simulink subsystem "Final_Project_DistHold_attempt_20260602_205044"  (R2024a)
settings: Solver=VariableStepAuto  StartTime=0.0  StopTime=10.0  RelTol=1e-3
values from neighbouring files (symbols this model uses):
  D = hypot(Ep(:,1)-Tp(:,1)',Ep(:,2)-Tp(:,2)')    [pp_compare_stage.m]    (also in pp_diag_path.m; pp_t09_clear.m = hypot(Ep(:,1)-Tperim(:,1)', Ep(:,2)-Tperim(:,2)'); pp_tune2.m)
undefined symbols (not defined in the file or in its folder): DiscIntNeverNeededParam, waypoint_const
libraries: CarMaker4SL x83, simulink x2
(part 5 of 5)

== matlab function Final_Project_DistHold_attempt_20260602_205044/Parking_system/MATLAB Function6 ==
  data: ego_x input; desired_ax output; ego_y input; ego_yaw input; ego_v input; start_point input; finish_point input; goal_yaw input; occ_map input; steer_fl output; steer_fr output; selector_ctrl output
function [desired_ax, steer_fl, steer_fr, selector_ctrl] = Parking(ego_x, ego_y, ego_yaw, ego_v, start_point, finish_point, goal_yaw, occ_map)
%PARKING  Self-contained version of the "MATLAB Function" block.
%   Source model : Models/Day4_5/Day4_5_Scenario_1.slx
%   Block path   : CarMaker/Subsystem/Day4 & 5/Scenario 1/MATLAB Function
%
%   The block body only calls the pp_* helper; this file additionally
%   bundles every pp_*.m it transitively depends on as local functions,
%   so it runs standalone without dev/day4_5/pp_*.m on the MATLAB path.
%
%   Bundled depQendencies (15): pp_parking, pp_ackermann, pp_angdiff, pp_axle_from_fr1, pp_cfg, pp_collision, pp_grid2world, pp_hybrid_astar, pp_pt_in_quad, pp_rect_corners, pp_reedsshepp, pp_rs_paths, pp_rs_sample, pp_track, pp_world2grid
[desired_ax, steer_fl, steer_fr, selector_ctrl] = pp_parking(ego_x, ego_y, ego_yaw, ego_v, start_point, finish_point, goal_yaw, occ_map);
end

% ========================================================================
%  Local dependency functions (bundled verbatim from dev/day4_5/pp_*.m).
%  Do not edit here; edit the pp_*.m sources and re-bundle.
% ========================================================================

function [desired_ax, steer_fl, steer_fr, selector_ctrl] = pp_parking(ego_x, ego_y, ego_yaw, ego_v, start_point, finish_point, goal_yaw, occ_map) %#ok<INUSD>
%#codegen
% PP_PARKING  Full precise-parking controller (M10 integration).
%   Supervisor: INIT -> PLAN (Hybrid A*+RS, once) -> TRACK (pure pursuit) ->
%   CORRECT (a few committed Reeds-Shepp corrective rounds, each tracked by
%   pp_track) -> PARKED. Using committed RS paths (fixed cusps) instead of
%   per-step RS feedback avoids gear-shift chatter on the real plant.
%   Gear FSM shifts only when (nearly) stopped. Longitudinal command is in the
%   DRIVING (gear) direction (CarMaker AccelCtrl convention) with an over-speed
%   guard. Ackermann splits the steer into L/R wheels.
%
%   Inputs (Car.Fr1 = rear-bumper center): ego_x,ego_y[m], ego_yaw, ego_v[m/s],
%   finish_point=[x y] (rear bumper), goal_yaw[rad], occ_map. start_point unused.
cfg = pp_cfg(); d_r = cfg.d_r; L = cfg.wheelbase; tw = cfg.track_f; MAXP = cfg.max_path;

persistent state PX PY PDIR NP seg gear replan nround
if isempty(state)
    state = uint8(0);
    PX = zeros(MAXP,1); PY = zeros(MAXP,1); PDIR = zeros(MAXP,1);
    NP = 0; seg = 1; gear = cfg.GEAR_P; replan = false; nround = 0;
end

[ex, ey] = pp_axle_from_fr1(ego_x, ego_y, ego_yaw, d_r); eth = ego_yaw;
gth = goal_yaw;
[gx, gy] = pp_axle_from_fr1(finish_point(1), finish_point(2), gth, d_r);

delta = 0.0; v_des = 0.0; hold = false;

switch state
    case uint8(0)                                       % INIT
        state = uint8(1); hold = true;

    case uint8(1)                                       % PLAN (one heavy step)
        [px, py, ~, pdir, np, ok] = pp_hybrid_astar(ex, ey, eth, gx, gy, gth, occ_map);
        if ok
            PX = px; PY = py; PDIR = pdir; NP = np; seg = 1; state = uint8(2);
        else
            state = uint8(4);
        end
        hold = true;

    case uint8(2)                                       % TRACK main path
        [delta, v_des, seg, done] = pp_track(ex, ey, eth, ego_v, PX, PY, PDIR, NP, seg, cfg);
        if done, state = uint8(3); replan = true; nround = 0; end

    case uint8(3)                                       % CORRECT (committed RS rounds)
        if replan
            [Tr, sLr, ~, okr] = pp_reedsshepp(ex, ey, eth, gx, gy, gth, cfg.Rmin);
            if okr
                [rx, ry, ~, rdir, rns] = pp_rs_sample(ex, ey, eth, Tr, sLr, cfg.Rmin, cfg.ds, MAXP);
                if rns >= 2
                    PX = rx; PY = ry; PDIR = rdir; NP = rns; seg = 1;
                    replan = false; nround = nround + 1;
                else
                    state = uint8(4);
                end
            else
                state = uint8(4);
            end
        end
        if state == uint8(3)
            [delta, v_des, seg, done] = pp_track(ex, ey, eth, ego_v, PX, PY, PDIR, NP, seg, cfg);
            if done
                if (hypot(gx-ex, gy-ey) < cfg.align_pos && abs(pp_angdiff(eth,gth)) < cfg.align_yaw) ...
                        || nround >= cfg.max_rounds
                    state = uint8(4);
                else
                    replan = true;                      % next committed round
                end
            end
        end

    otherwise                                           % PARKED
        hold = true;
end
if state == uint8(4), hold = true; end

% --- outputs: gear FSM + longitudinal (driving-dir) + Ackermann ---
if hold
    selector_ctrl = cfg.GEAR_P;
    desired_ax    = -1.0;
    steer_fl      = 0.0; steer_fr = 0.0;
else
    if abs(ego_v) < cfg.v_stop                          % shift only when ~stopped
        if v_des > 0.02
            gear = cfg.GEAR_D;
        elseif v_des < -0.02
            gear = cfg.GEAR_R;
        end
    end
    selector_ctrl = gear;
    % CarMaker AccelCtrl.DesiredAx = GEAR-DIRECTION acceleration demand (CONFIRMED by
    % per-gear regression of the logs: in D +DesiredAx -> +x accel (slope +0.84); in R
    % +DesiredAx -> -x accel (slope -0.90)). So +DesiredAx = gas in the CURRENT GEAR
    % direction (forward in D, BACKWARD in R); -DesiredAx = brake. PRIMARY control is this
    % gear-direction speed regulation toward |v_des|, tracked by the vehicle's AccelCtrl PI
    % (tuned in the .car: higher i compensates the reverse idle-creep). Reverse uses a LOW
    % target speed (cfg.v_rev). The over-target branch is only a SAFETY NET (large margin)
    % in case the PI lags -- it should rarely fire once the PI holds the low reverse speed.
    if gear == cfg.GEAR_R, gdir = -1.0; else, gdir = 1.0; end
    v_drive = gdir*ego_v;                                  % speed in the gear (driving) direction
    desired_ax = cfg.kp_v*(abs(v_des) - v_drive);         % + = gas (gear dir), - = brake
    desired_ax = max(min(desired_ax, cfg.ax_max), -cfg.ax_max);
    if v_drive > cfg.v_emax                                % SAFETY NET: genuine runaway only (PI now
        desired_ax = -cfg.ax_brake;                       % regulates normal speed; no mid-maneuver stops)
    end
    [steer_fl, steer_fr] = pp_ackermann(delta, L, tw);
end
end

function [dL, dR] = pp_ackermann(delta, L, tw)
%#codegen
% PP_ACKERMANN  Left/right front road-wheel angles from a single bicycle steer.
%   delta : bicycle (center) steer angle [rad]; L : wheelbase; tw : front track.
%   Inner wheel steers more than the outer (true Ackermann geometry).
if abs(delta) < 1e-4
    dL = 0.0; dR = 0.0;
    return;
end
R  = L / tan(delta);            % signed turn radius at rear-axle center (+ = left)
dL = atan(L / (R - tw/2));      % left  front wheel
dR = atan(L / (R + tw/2));      % right front wheel
end

function d = pp_angdiff(a, b)
%#codegen
% PP_ANGDIFF  Smallest signed angle a-b wrapped to [-pi, pi].
d = mod(a - b + pi, 2*pi) - pi;
end

function [xa, ya] = pp_axle_from_fr1(x, y, yaw, d_r)
%#codegen
% PP_AXLE_FROM_FR1  Rear-axle position from Fr1 (rear-bumper) pose.
%   Rear axle sits d_r ahead of Fr1 along the heading.
xa = x + d_r*cos(yaw);
ya = y + d_r*sin(yaw);
end

function cfg = pp_cfg()
%#codegen
% PP_CFG  Configuration for the Day4/5 precise-parking controller (Kia_EV6).
%   Geometry from Data/Vehicle/Kia_EV6 (Vehicle.OuterSkin & wheel positions).
%
%   Pose convention (CarMaker): Car.Fr1 origin = REAR-BUMPER center on the road,
%   X forward, Y left, yaw = Car.Fr1.rz [rad]. Same convention for the mission
%   goal pose and every obstacle coordinate. Internal planning/tracking uses the
%   REAR AXLE, d_r ahead of Fr1:  rear_axle = Fr1 + d_r*[cos(yaw) sin(yaw)].
%
%   CODEGEN NOTE: build every struct field from LOCAL variables / literals only.
%   Never read a cfg field while still constructing cfg.

% --- local geometry constants (Kia_EV6) -----------------------------------
veh_L     = 4.68;
veh_W     = 1.88;
wheelbase = 2.90;
d_r       = 0.95;
delta_max = 30*pi/180;

% --- vehicle ---------------------------------------------------------------
cfg.veh_L       = veh_L;
cfg.veh_W       = veh_W;
cfg.veh_halfW   = veh_W/2;
cfg.wheelbase   = wheelbase;
cfg.track_f     = 1.624;                  % front track width [m] (wheels at y=+-0.812)
cfg.d_r         = d_r;
cfg.foot_ahead  = veh_L - d_r;            % rear-axle -> front bumper [m] = 3.73
cfg.foot_behind = d_r;                    % rear-axle -> rear bumper  [m] = 0.95
cfg.delta_max   = delta_max;
cfg.Rmin        = wheelbase / tan(delta_max);

% --- obstacle vehicle (IPG_CompanyCar_2018_Blue) ---------------------------
cfg.obs_L       = 4.47;
cfg.obs_W       = 1.97;
cfg.holdout     = 14;                     % pp_obstacles row kept FREE as the parking
                                          %   target (held-out car). 14 = T13. 0 = none.

% --- occupancy grid --------------------------------------------------------
cfg.n           = 200;                    % cells/side (occ_map [200 200]) -- keep 200: EML occ port is fixed
cfg.margin      = 0.30;                   % obstacle footprint safety inflation [m] (buffer for tracking error)
cfg.bounds      = [-5 48 -45.5 6];        % world planning rect [xmin xmax ymin ymax] = lot + NORTH entrance approach
                                          %   (res 53/200=0.265 x 51.5/200=0.258 m)
cfg.lot         = [2 48 -45.5 -3];        % drivable parking-lot rectangle [xmin xmax ymin ymax] (carved FREE by pp_generate_map)
cfg.edge_margin = 0.20;                    % safety margin inset from the drivable-region boundary (lot edges + corridor walls) [m]
cfg.wall_cells  = 1;                      % occupied border-ring thickness [cells]

% --- Hybrid A* planner -----------------------------------------------------
cfg.plan_res    = 0.5;                    % closed-set position resolution [m]
cfg.nxc         = 106;                    % closed-set X bins  ~ (bounds_x)/plan_res = 53/0.5
cfg.nyc         = 103;                    % closed-set Y bins  ~ (bounds_y)/plan_res = 51.5/0.5
cfg.nth         = 72;                     % heading bins (5 deg)
cfg.ds          = 0.6;                    % motion step (arc length) [m]
cfg.n_steer     = 5;                      % steering samples (odd, symmetric)
cfg.max_nodes   = 60000;                  % expansion / node cap
cfg.max_path    = 2000;                   % max stored path points
cfg.pos_tol     = 0.7;                    % planner goal position tol [m] (M9 refines)
cfg.yaw_tol     = 12*pi/180;              % planner goal heading tol [rad]
cfg.w_rev       = 2.0;                    % reverse cost multiplier
cfg.w_switch    = 2.0;                    % direction-change penalty [~m]
cfg.w_steer     = 0.3;                    % steering magnitude penalty
cfg.h_weight    = 1.2;                    % heuristic weight (>=1 speeds search)
cfg.rs_shot_dist = 15.0;                  % try RS one-shot to goal within this dist [m]
cfg.rs_heur_dist = 25.0;                  % use RS (vs Euclidean) heuristic within [m]

% --- M7 path tracking + longitudinal control -------------------------------
cfg.Ld          = 1.5;                    % (legacy) nominal lookahead [m]
cfg.Ld_min      = 0.5;                    % min lookahead (tight low-speed tracking) [m]
cfg.Ld_max      = 1.8;                    % max lookahead [m]
cfg.kld         = 1.2;                    % lookahead gain vs |speed| (Ld = Ld_min + kld*|v|)
cfg.v_fwd       = 1.0;                    % forward cruise speed [m/s] (faster approach)
cfg.v_rev       = 0.2;                    % reverse cruise speed [m/s] (known-good; speed-up revisited separately)
cfg.v_creep     = 0.10;                   % min creep speed while cruising [m/s]
cfg.v_stop      = 0.10;                   % treated as stopped [m/s]
cfg.kp_v        = 0.6;                    % longitudinal P gain (outer speed loop)
cfg.ax_max      = 0.6;                    % accel/brake command limit [m/s^2]
cfg.ax_min      = -1.5;                   % emergency decel/brake limit [m/s^2]
cfg.v_emax      = 1.2;                    % over-speed guard -> emergency brake [m/s]
cfg.v_obrake    = 0.40;                   % SAFETY-NET margin over target -> hard brake [m/s] (PI handles normal regulation)
cfg.ax_brake    = 1.5;                    % safety-net brake demand magnitude [m/s^2] (gear-dir: -ve = brake)
cfg.d_slow      = 5.0;                    % slow-down distance before cusp/goal [m] (weak brake -> decelerate early)
cfg.cusp_reach  = 0.30;                   % distance to register a cusp reached [m]
cfg.goal_reach  = 0.08;                   % path-end position tol [m]
cfg.max_rounds  = 4;                      % max RS corrective rounds in ALIGN (few shifts)

% --- M9 precise pose alignment (Astolfi pose regulation) -------------------
cfg.align_dist  = 3.0;                    % switch to alignment within this dist [m]
cfg.align_pos   = 0.08;                   % alignment done position tol [m]
cfg.align_yaw   = 2*pi/180;               % alignment done heading tol [rad]
cfg.v_align     = 0.3;                    % alignment creep speed [m/s]
cfg.v_align_min = 0.15;                   % min alignment creep speed [m/s]
cfg.kr          = 0.5;                    % Astolfi rho gain (approach)
cfg.ka          = 1.5;                    % Astolfi alpha gain (bearing)
cfg.kb          = -0.5;                   % Astolfi beta gain (final heading, <0)

% --- CarMaker gear selector enum (include/Vehicle.h) -----------------------
cfg.GEAR_P      = -9;
cfg.GEAR_R      = -1;
cfg.GEAR_N      = 0;
cfg.GEAR_D      = 1;
end

function tf = pp_collision(map, x, y, yaw, ahead, behind, halfw, b, n)
%#codegen
% PP_COLLISION  True if the oriented footprint at pose (x,y,yaw) overlaps any
%   occupied cell (map > 0). Pose is the REAR-AXLE reference; the footprint
%   spans [-behind,+ahead] x [-halfw,+halfw]. Scans the footprint bounding box.
c = pp_rect_corners(x, y, yaw, ahead, behind, halfw);
ixv = zeros(1, 4); iyv = zeros(1, 4);
for k = 1:4
    [ixv(k), iyv(k)] = pp_world2grid(c(k,1), c(k,2), b, n);
end
imin = max(min(ixv), 1); imax = min(max(ixv), n);
jmin = max(min(iyv), 1); jmax = min(max(iyv), n);
tf = false;
for ix = imin:imax
    for iy = jmin:jmax
        if map(iy, ix) > 0
            [cx, cy] = pp_grid2world(ix, iy, b, n);
            if pp_pt_in_quad(cx, cy, c)
                tf = true;
                return;
            end
        end
    end
end
end

function [x, y] = pp_grid2world(ix, iy, b, n)
%#codegen
% PP_GRID2WORLD  1-based grid indices -> world coordinates of the CELL CENTER.
%   b = [xmin xmax ymin ymax], n = cells per side.
resx = (b(2) - b(1)) / n;
resy = (b(4) - b(3)) / n;
x = b(1) + (ix - 0.5) * resx;
y = b(3) + (iy - 0.5) * resy;
end

function [px, py, pth, pdir, np, ok] = pp_hybrid_astar(xs, ys, ths, xg, yg, thg, occ_map)
%#codegen
% PP_HYBRID_ASTAR  Hybrid A* parking planner with Reeds-Shepp (REAR-AXLE frame).
%   In : start (xs,ys,ths), goal (xg,yg,thg) [rad], occ_map (n x n, 1=occupied).
%   Out: px,py,pth (max_path x1); pdir (+1 fwd / -1 rev per point); np count; ok.
%   Bicycle fwd/rev primitives + footprint collision; open=min-heap on f=g+h;
%   closed=best-g per (cell,heading). Heuristic = Reeds-Shepp length near goal
%   (Euclidean far). RS one-shot connects to the EXACT goal pose when close.

cfg = pp_cfg();
b = cfg.bounds; n = cfg.n;
plan_res = cfg.plan_res; nxc = cfg.nxc; nyc = cfg.nyc; nth = cfg.nth;
ds = cfg.ds; Lwb = cfg.wheelbase; dmax = cfg.delta_max; Rmin = cfg.Rmin;
ahead = cfg.foot_ahead; behind = cfg.foot_behind; halfw = cfg.veh_halfW;
MAXN = cfg.max_nodes; MAXP = cfg.max_path; ns = cfg.n_steer; hw = cfg.h_weight;
rs_shot = cfg.rs_shot_dist; rs_heur = cfg.rs_heur_dist;
dth_bin = 2*pi/nth;

% steering samples (symmetric about 0)
steer = zeros(1, ns);
for i = 1:ns
    steer(i) = -dmax + (i-1)*(2*dmax/(ns-1));
end

% node + heap + closed storage
NX = zeros(MAXN,1); NY = zeros(MAXN,1); NT = zeros(MAXN,1);
NG = inf(MAXN,1);   NPar = zeros(MAXN,1); NDir = zeros(MAXN,1);
HID = zeros(MAXN,1); HF = inf(MAXN,1); hn = 0;
gbest = inf(nxc, nyc, nth);

% outputs + RS one-shot buffer
px = zeros(MAXP,1); py = zeros(MAXP,1); pth = zeros(MAXP,1); pdir = zeros(MAXP,1);
np = 0; ok = false;
rsx = zeros(MAXP,1); rsy = zeros(MAXP,1); rsth = zeros(MAXP,1); rsdir = zeros(MAXP,1);
rsn = 0; viars = false;

% seed start node
ncount = 1;
NX(1) = xs; NY(1) = ys; NT(1) = ths; NG(1) = 0; NPar(1) = 0; NDir(1) = 0;
six = min(max(floor((xs-b(1))/plan_res)+1,1),nxc);
siy = min(max(floor((ys-b(3))/plan_res)+1,1),nyc);
sit = mod(floor(mod(ths,2*pi)/dth_bin),nth)+1;
gbest(six,siy,sit) = 0;
hn = hn + 1; HID(hn) = 1;
HF(hn) = hw*heur_(xs, ys, ths, xg, yg, thg, Rmin, rs_heur);

goalid = 0; iters = 0;
while hn > 0 && iters < MAXN
    iters = iters + 1;

    % --- heap pop (min f) ---
    cur = HID(1);
    HID(1) = HID(hn); HF(1) = HF(hn); hn = hn - 1;
    hc = 1;
    while true
        hl = 2*hc; hr = 2*hc+1; sm = hc;
        if hl <= hn && HF(hl) < HF(sm), sm = hl; end
        if hr <= hn && HF(hr) < HF(sm), sm = hr; end
        if sm == hc, break; end
        tf = HF(sm); HF(sm) = HF(hc); HF(hc) = tf;
        tk = HID(sm); HID(sm) = HID(hc); HID(hc) = tk;
        hc = sm;
    end

    cx = NX(cur); cy = NY(cur); cth = NT(cur); cg = NG(cur); cdir = NDir(cur);

    % --- tol goal test (fallback) ---
    if abs(cx-xg) < cfg.pos_tol && abs(cy-yg) < cfg.pos_tol && ...
            abs(pp_angdiff(cth,thg)) < cfg.yaw_tol
        goalid = cur; ok = true; break;
    end

    % --- Reeds-Shepp one-shot to exact goal (when close) ---
    if hypot(cx-xg, cy-yg) < rs_shot
        [Tg, segLg, ~, okg] = pp_reedsshepp(cx, cy, cth, xg, yg, thg, Rmin);
        if okg
            [tx, ty, tth, tdir, tn] = pp_rs_sample(cx, cy, cth, Tg, segLg, Rmin, ds, MAXP);
            free = true;
            for sidx = 1:tn
                if pp_collision(occ_map, tx(sidx),ty(sidx),tth(sidx), ahead,behind,halfw, b, n)
                    free = false; break;
                end
            end
            if free
                goalid = cur; ok = true; viars = true; rsn = tn;
                for sidx = 1:tn
                    rsx(sidx)=tx(sidx); rsy(sidx)=ty(sidx); rsth(sidx)=tth(sidx); rsdir(sidx)=tdir(sidx);
                end
                break;
            end
        end
    end

    % --- expand successors (2 directions x ns steers) ---
    for di = 1:2
        if di == 1, dir = 1.0; else, dir = -1.0; end
        sgn = dir*ds;
        for si = 1:ns
            st = steer(si);
            if abs(st) < 1e-6
                nthp = cth;
                nxp = cx + sgn*cos(cth);  nyp = cy + sgn*sin(cth);
                mthp = cth;
                mxp = cx + 0.5*sgn*cos(cth);  myp = cy + 0.5*sgn*sin(cth);
            else
                R = Lwb/tan(st);
                nthp = cth + sgn/R;
                nxp = cx + R*(sin(nthp)-sin(cth));
                nyp = cy - R*(cos(nthp)-cos(cth));
                mthp = cth + 0.5*sgn/R;
                mxp = cx + R*(sin(mthp)-sin(cth));
                myp = cy - R*(cos(mthp)-cos(cth));
            end

            if pp_collision(occ_map, mxp,myp,mthp, ahead,behind,halfw, b, n), continue; end
            if pp_collision(occ_map, nxp,nyp,nthp, ahead,behind,halfw, b, n), continue; end

            stepc = ds;
            if dir < 0, stepc = stepc + ds*(cfg.w_rev-1); end
            if cdir ~= 0 && dir ~= cdir, stepc = stepc + cfg.w_switch; end
            stepc = stepc + cfg.w_steer*abs(st);
            ng = cg + stepc;

            kix = min(max(floor((nxp-b(1))/plan_res)+1,1),nxc);
            kiy = min(max(floor((nyp-b(3))/plan_res)+1,1),nyc);
            kit = mod(floor(mod(nthp,2*pi)/dth_bin),nth)+1;

            if ng < gbest(kix,kiy,kit) && ncount < MAXN
                gbest(kix,kiy,kit) = ng;
                ncount = ncount + 1;
                NX(ncount)=nxp; NY(ncount)=nyp; NT(ncount)=nthp;
                NG(ncount)=ng;  NPar(ncount)=cur; NDir(ncount)=dir;
                fval = ng + hw*heur_(nxp, nyp, nthp, xg, yg, thg, Rmin, rs_heur);
                hn = hn + 1; HID(hn) = ncount; HF(hn) = fval;
                hc = hn;
                while hc > 1
                    hp = floor(hc/2);
                    if HF(hp) <= HF(hc), break; end
                    tf = HF(hp); HF(hp) = HF(hc); HF(hc) = tf;
                    tk = HID(hp); HID(hp) = HID(hc); HID(hc) = tk;
                    hc = hp;
                end
            end
        end
    end
end

% --- reconstruct: Hybrid path (start -> goalid), then append RS one-shot ---
if ok && goalid > 0
    tmpx = zeros(MAXP,1); tmpy = zeros(MAXP,1); tmpt = zeros(MAXP,1); tmpd = zeros(MAXP,1);
    cntr = 0; node = goalid;
    while node ~= 0 && cntr < MAXP
        cntr = cntr + 1;
        tmpx(cntr)=NX(node); tmpy(cntr)=NY(node); tmpt(cntr)=NT(node); tmpd(cntr)=NDir(node);
        node = NPar(node);
    end
    np = cntr;
    for i = 1:cntr
        j = cntr - i + 1;
        px(i)=tmpx(j); py(i)=tmpy(j); pth(i)=tmpt(j); pdir(i)=tmpd(j);
    end
    if cntr >= 2, pdir(1) = pdir(2); end
    if viars
        for sidx = 2:rsn                       % skip RS sample 1 (== node, already added)
            if np >= MAXP, break; end
            np = np + 1;
            px(np)=rsx(sidx); py(np)=rsy(sidx); pth(np)=rsth(sidx); pdir(np)=rsdir(sidx);
        end
    end
end
end

% ===== heuristic: RS length near goal, Euclidean far ======================
function h = heur_(x, y, th, xg, yg, thg, Rmin, rs_heur)
%#codegen
eu = hypot(x-xg, y-yg);
if eu < rs_heur
    [~, ~, Lr, okr] = pp_reedsshepp(x, y, th, xg, yg, thg, Rmin);
    if okr && Lr > eu, h = Lr; else, h = eu; end
else
    h = eu;
end
end

function tf = pp_pt_in_quad(px, py, c)
%#codegen
% PP_PT_IN_QUAD  True if point (px,py) lies inside the convex quad c (4-by-2).
%   Winding-agnostic: inside iff the point is on the same side of all 4 edges.
s = zeros(1, 4);
for k = 1:4
    k2 = mod(k, 4) + 1;
    ex = c(k2,1) - c(k,1);
    ey = c(k2,2) - c(k,2);
    s(k) = ex*(py - c(k,2)) - ey*(px - c(k,1));
end
tf = all(s >= -1e-9) || all(s <= 1e-9);
end

function c = pp_rect_corners(x, y, yaw, ahead, behind, halfw)
%#codegen
% PP_RECT_CORNERS  World corners (4-by-2) of an oriented rectangle.
%   Local frame: X forward, Y left. Rectangle spans X in [-behind, +ahead]
%   and Y in [-halfw, +halfw], placed at pose (x, y, yaw).
%   Corner order: front-left, front-right, rear-right, rear-left (clockwise).
co = cos(yaw); si = sin(yaw);
lx = [ahead,  ahead, -behind, -behind];
ly = [halfw, -halfw, -halfw,   halfw];
c = zeros(4, 2);
for k = 1:4
    c(k,1) = x + co*lx(k) - si*ly(k);
    c(k,2) = y + si*lx(k) + co*ly(k);
end
end

function [T, segLen, Ltot, ok] = pp_reedsshepp(x0, y0, th0, x1, y1, th1, Rmin)
%#codegen
% PP_REEDSSHEPP  Shortest Reeds-Shepp word (CSC+CCC set) between two poses.
%   In : start (x0,y0,th0), goal (x1,y1,th1) [rad], turning radius Rmin [m].
%   Out: T(1x3) segment types (1=L,2=S,3=R); segLen(1x3) signed arc lengths [m]
%        (sign = drive direction); Ltot total length [m]; ok success flag.
dx = x1 - x0;  dy = y1 - y0;
c = cos(th0);  s = sin(th0);
xn = ( c*dx + s*dy) / Rmin;          % goal in start frame, scaled to unit radius
yn = (-s*dx + c*dy) / Rmin;
phi = pp_angdiff(th1, th0);

[T, Lr, Ltot_r, ok] = pp_rs_paths(xn, yn, phi);
segLen = Lr * Rmin;
Ltot   = Ltot_r * Rmin;
end

function [T, L, Ltot, ok] = pp_rs_paths(x, y, phi)
%#codegen
% PP_RS_PATHS  Shortest Reeds-Shepp word for a unit-radius normalized goal
%   (x,y,phi) expressed in the start frame. Covers the CSC + CCC families
%   (LSL,LSR,RSR,RSL,LRL,RLR) via the 3 base words x {id, time-flip, reflect,
%   both} = 12 candidates. Returns:
%     T    : 1x3 segment types (1=L, 2=S, 3=R)
%     L    : 1x3 signed segment lengths in RADIUS units (sign = drive direction)
%     Ltot : total |length| (radius units)
%     ok   : a valid word was found
best = inf;
T = [1 2 1]; L = [0 0 0]; ok = false;

for base = 1:3                 % 1=LSL, 2=LSR, 3=LRL
    for sym = 1:4              % 1=identity, 2=time-flip, 3=reflect, 4=both
        xx = x; yy = y; pp = phi;
        if sym == 2,  xx = -x; yy =  y; pp = -phi; end   % time-flip
        if sym == 3,  xx =  x; yy = -y; pp = -phi; end   % reflect
        if sym == 4,  xx = -x; yy = -y; pp =  phi; end   % both

        [okk, t, u, v] = rs_base(base, xx, yy, pp);
        if ~okk, continue; end

        lens = [t, u, v];
        if sym == 2 || sym == 4, lens = -lens; end        % time-flip negates lengths

        ct = [1 2 1];
        if base == 2, ct = [1 2 3]; elseif base == 3, ct = [1 3 1]; end
        if sym == 3 || sym == 4                           % reflect swaps L<->R
            ct = swapLR(ct);
        end

        tot = abs(lens(1)) + abs(lens(2)) + abs(lens(3));
        if tot < best
            best = tot; T = ct; L = lens; ok = true;
        end
    end
end
Ltot = best;
if ~ok, Ltot = 0; end
end

% ===== base words (PythonRobotics formulation, unit radius) ================
function [ok, t, u, v] = rs_base(base, x, y, phi)
%#codegen
if base == 1
    [ok, t, u, v] = rs_LSL(x, y, phi);
elseif base == 2
    [ok, t, u, v] = rs_LSR(x, y, phi);
else
    [ok, t, u, v] = rs_LRL(x, y, phi);
end
end

function [ok, t, u, v] = rs_LSL(x, y, phi)
%#codegen
ok = false; v = 0;
[u, t] = rs_polar(x - sin(phi), y - 1 + cos(phi));
if t >= 0
    v = rs_mod2pi(phi - t);
    if v >= 0, ok = true; end
end
end

function [ok, t, u, v] = rs_LSR(x, y, phi)
%#codegen
ok = false; t = 0; u = 0; v = 0;
[u1, t1] = rs_polar(x + sin(phi), y - 1 - cos(phi));
u1sq = u1*u1;
if u1sq >= 4
    u = sqrt(u1sq - 4);
    theta = atan2(2.0, u);
    t = rs_mod2pi(t1 + theta);
    v = rs_mod2pi(t - phi);
    if t >= 0 && v >= 0, ok = true; end
end
end

function [ok, t, u, v] = rs_LRL(x, y, phi)
%#codegen
ok = false; t = 0; u = 0; v = 0;
[u1, t1] = rs_polar(x - sin(phi), y - 1 + cos(phi));
if u1 <= 4
    u = -2*asin(u1/4);
    t = rs_mod2pi(t1 + 0.5*u + pi);
    v = rs_mod2pi(phi - t + u);
    if t >= 0 && u <= 0, ok = true; end
end
end

% ===== helpers =============================================================
function [r, th] = rs_polar(a, b)
%#codegen
r = hypot(a, b);
th = atan2(b, a);
end

function v = rs_mod2pi(x)
%#codegen
v = mod(x, 2*pi);
if v > pi, v = v - 2*pi; end
end

function c = swapLR(c)
%#codegen
for k = 1:3
    if c(k) == 1, c(k) = 3; elseif c(k) == 3, c(k) = 1; end
end
end

function [sx, sy, sth, sdir, ns] = pp_rs_sample(x0, y0, th0, T, segLen, Rmin, ds, MAXP)
%#codegen
% PP_RS_SAMPLE  Sample a Reeds-Shepp path into poses for collision checks/output.
%   T(1x3) types (1=L,2=S,3=R), segLen(1x3) signed arc lengths [m].
%   Returns poses sx,sy,sth (MAXP x1), per-point direction sdir (+1/-1), ns count.
sx = zeros(MAXP,1); sy = zeros(MAXP,1); sth = zeros(MAXP,1); sdir = zeros(MAXP,1);
x = x0; y = y0; th = th0;
k = 1; sx(1) = x; sy(1) = y; sth(1) = th; sdir(1) = sign_nz(segLen(1));

for i = 1:3
    Li = segLen(i);
    if abs(Li) < 1e-9, continue; end
    dirn = sign_nz(Li);
    if T(i) == 1
        kappa =  1/Rmin;
    elseif T(i) == 3
        kappa = -1/Rmin;
    else
        kappa = 0;
    end
    dist  = abs(Li);
    steps = max(1, ceil(dist/ds));
    step  = dist/steps;
    for j = 1:steps
        if k >= MAXP, break; end
        sgn = dirn*step;
        if kappa == 0
            x = x + sgn*cos(th);
            y = y + sgn*sin(th);
        else
            th2 = th + sgn*kappa;
            x = x + (sin(th2) - sin(th))/kappa;
            y = y - (cos(th2) - cos(th))/kappa;
            th = th2;
        end
        k = k + 1;
        sx(k) = x; sy(k) = y; sth(k) = th; sdir(k) = dirn;
    end
end
ns = k;
end

function s = sign_nz(v)
%#codegen
if v < 0, s = -1.0; else, s = 1.0; end
end

function [delta, v_des, seg, done] = pp_track(ax, ay, ath, v, PX, PY, PDIR, NP, seg, cfg)
%#codegen
% PP_TRACK  Reverse-aware pure-pursuit path tracker (REAR-AXLE frame).
%   In : ego rear-axle pose (ax,ay,ath), signed speed v, path PX,PY,PDIR(1..NP),
%        current segment index seg, cfg.
%   Out: delta (front road-wheel steer [rad]); v_des (signed target speed [m/s]);
%        seg (advanced, monotonic); done (goal reached).
%   Stays within the current-direction segment (no jumps across cusps), forces a
%   full stop at each cusp before switching direction, and stops at the goal.
L = cfg.wheelbase;
delta = 0; v_des = 0; done = false;
if NP < 2, done = true; return; end
if seg < 1, seg = 1; end
if seg > NP, seg = NP; end

dir = PDIR(seg); if dir == 0, dir = 1; end

% end index of the current-direction segment (cusp = jc, or NP if last)
jc = NP;
for i = seg:NP
    if PDIR(i) ~= dir, jc = i-1; break; end
end
if jc < seg, jc = seg; end

% windowed closest point, clamped to the current segment [seg, jc]
W = 12; hi = min(seg + W, jc);
ci = seg; bestd = inf;
for i = seg:hi
    dxi = PX(i)-ax; dyi = PY(i)-ay;
    di = dxi*dxi + dyi*dyi;
    if di < bestd, bestd = di; ci = i; end
end
seg = ci;

% remaining arc to segment end
remain = 0;
for i = ci:NP-1
    if i >= jc, break; end
    remain = remain + hypot(PX(i+1)-PX(i), PY(i+1)-PY(i));
end
% speed-adaptive lookahead (short at low speed -> tight tracking), capped by remain
Ldspeed = cfg.Ld_min + cfg.kld*abs(v);
Ldeff = min([Ldspeed, cfg.Ld_max, max(remain, cfg.Ld_min)]);
if Ldeff < cfg.Ld_min, Ldeff = cfg.Ld_min; end

% lookahead target within [ci, jc]
ti = min(ci+1, NP); acc = 0; i = ci;
while i < jc && acc < Ldeff
    acc = acc + hypot(PX(i+1)-PX(i), PY(i+1)-PY(i));
    ti = i + 1; i = i + 1;
end
xt = PX(ti); yt = PY(ti);

% pure-pursuit steering (reverse-aware)
bea = atan2(yt-ay, xt-ax);
if dir < 0, head = ath + pi; else, head = ath; end
alpha = pp_angdiff(bea, head);
Ldact = max(hypot(xt-ax, yt-ay), 0.3);
delta = atan2(2*L*sin(alpha), Ldact);
if dir < 0, delta = -delta; end
delta = max(min(delta, cfg.delta_max), -cfg.delta_max);

% speed target: cruise (creep floor), slow approaching the segment end / goal
d_cusp = hypot(PX(jc)-ax, PY(jc)-ay);
d_goal = hypot(PX(NP)-ax, PY(NP)-ay);
dmin = min(d_cusp, d_goal);
if dir > 0, vmax = cfg.v_fwd; else, vmax = cfg.v_rev; end   % faster fwd, slower rev
vmag = max(cfg.v_creep, vmax * min(1.0, dmin/cfg.d_slow));
v_des = dir * vmag;

% stop logic: full stop at a cusp before switching dir, or at the goal
if jc < NP
    if ci >= jc || d_cusp < cfg.cusp_reach
        v_des = 0;
        if abs(v) < cfg.v_stop, seg = jc + 1; end          % switch into next segment
    end
else
    % longitudinal progress toward the final point (handles overshoot)
    p2 = max(NP-1, 1);
    ux = PX(NP)-PX(p2); uy = PY(NP)-PY(p2);
    un = hypot(ux, uy); if un < 1e-6, un = 1; end
    sprog = ((PX(NP)-ax)*ux + (PY(NP)-ay)*uy) / un;
    if d_goal < cfg.goal_reach || sprog <= 0
        v_des = 0;
        if abs(v) < cfg.v_stop, done = true; delta = 0; end
    end
end
end

function [ix, iy] = pp_world2grid(x, y, b, n)
%#codegen
% PP_WORLD2GRID  World (x,y) -> 1-based grid indices (ix along X/col, iy along Y/row).
%   b = [xmin xmax ymin ymax], n = cells per side. Indices clamped to [1,n].
resx = (b(2) - b(1)) / n;
resy = (b(4) - b(3)) / n;
ix = floor((x - b(1)) / resx) + 1;
iy = floor((y - b(3)) / resy) + 1;
ix = min(max(ix, 1), n);
iy = min(max(iy, 1), n);
end
